simulink model "model19a"  (Simulink 9.3)
settings: Solver=ode8  StartTime=0.0  StopTime=10  FixedStep=1e-4  RelTol=1e-3
undefined symbols (not defined in the file): a_vect, b_vect, fm_vect, fp, gm_vect, r_vect, s_vect, t_vect, Ts
settings Model: Creator=lukze  LastModifiedBy=Lukáš Zezula
settings DataIOCC: SaveFormat=Dataset  SignalLoggingSaveFormat=Dataset  ReturnWorkspaceOutputs=on
settings OptimizationCC: LifeSpan=auto
settings DebuggingCC: UnderspecifiedInitializationDetection=Simplified  MergeDetectMultiDrivingBlocksExec=error  FcnCallInpInsideContextMsg=error  SFUnexpectedBacktrackingDiag=error  SFNoUnconditionalDefaultTransitionDiag=error  SFExecutionAtInitializationDiag=warning  ArithmeticOperatorsInVariantConditions=error
settings HardwareCC: ProdBitPerPointer=64  ProdBitPerSizeT=64  ProdBitPerPtrDiffT=64  ProdLargestAtomicFloat=Float  ProdIntDivRoundTo=Zero  ProdEndianess=LittleEndian  ProdWordSize=64  ProdHWDeviceType=Intel->x86-64 (Windows64)
settings ModelReferenceCC: PropagateSignalLabelsOutOfModel=on
settings SFSimCC: SimUseLocalCustomCode=on
settings RTWCC: RTWUseLocalCustomCode=on
settings CodeAppCC: StateflowObjectComments=off
settings GRTTargetCC: TargetLangStandard=C99 (ISO)  CombineOutputUpdateFcns=on  GRTInterface=off
settings ConfigComp: CovMetricSettings=dwe  CovSaveCumulativeToWorkspaceVar=off  CovSaveSingleToWorkspaceVar=off  CovExternalEMLEnable=on

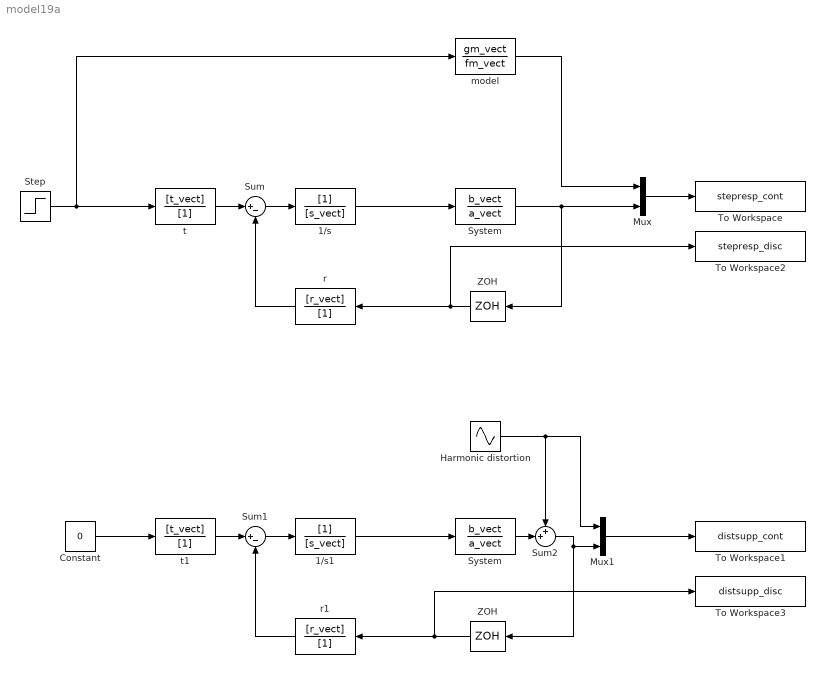
== system model19a ==
  " System " : TransferFcn  Numerator=b_vect  Denominator=a_vect
  1/s : DiscreteFilter  Denominator=[s_vect]  SampleTime=Ts
  1/s1 : DiscreteFilter  Denominator=[s_vect]  SampleTime=Ts
  Constant : Constant  Value=0  SampleTime=-1
  Harmonic distortion : Sin  Frequency=2*pi*fp  SampleTime=1e-4
  Mux : Mux  Inputs=2
  Mux1 : Mux  Inputs=2
  Step : Step  Time=0  SampleTime=1e-4
  Sum : Sum  Inputs=|+-
  Sum1 : Sum  Inputs=|+-
  Sum2 : Sum  Inputs=++|
  System : TransferFcn  Numerator=b_vect  Denominator=a_vect
  To Workspace : ToWorkspace  VariableName=stepresp_cont  SaveFormat=Timeseries  SampleTime=-1
  To Workspace1 : ToWorkspace  VariableName=distsupp_cont  SaveFormat=Timeseries  SampleTime=-1
  To Workspace2 : ToWorkspace  VariableName=stepresp_disc  SaveFormat=Timeseries  SampleTime=-1
  To Workspace3 : ToWorkspace  VariableName=distsupp_disc  SaveFormat=Timeseries  SampleTime=-1
  ZOH : ZeroOrderHold  SampleTime=Ts
  "ZOH " : ZeroOrderHold  SampleTime=Ts
  model : TransferFcn  Numerator=gm_vect  Denominator=fm_vect
  r : DiscreteFilter  Numerator=[r_vect]  Denominator=[1]  SampleTime=Ts
  r1 : DiscreteFilter  Numerator=[r_vect]  Denominator=[1]  SampleTime=Ts
  t : DiscreteFilter  Numerator=[t_vect]  Denominator=[1]  SampleTime=Ts
  t1 : DiscreteFilter  Numerator=[t_vect]  Denominator=[1]  SampleTime=Ts
  wires:
  t/1 -> Sum/1
  r/1 -> Sum/2
  Sum/1 -> 1/s/1
  1/s/1 -> System/1
  ZOH/1 -> To Workspace2/1, r/1
  System/1 -> Mux/2, ZOH/1
  Mux/1 -> To Workspace/1
  model/1 -> Mux/1
  Constant/1 -> t1/1
  1/s1/1 -> " System "/1
  "ZOH "/1 -> To Workspace3/1, r1/1
  " System "/1 -> Sum2/2
  Harmonic distortion/1 -> Mux1/1, Sum2/1
  Sum2/1 -> "ZOH "/1, Mux1/2
  Mux1/1 -> To Workspace1/1
  r1/1 -> Sum1/2
  t1/1 -> Sum1/1
  Sum1/1 -> 1/s1/1
  Step/1 -> t/1, model/1
